simulink model "MSD_4"  (R2021b)
settings: Solver=ode4  StartTime=0.0  StopTime=10.0  FixedStep=0.1  RelTol=1e-3
values from neighbouring files (symbols this model uses):
  A = [0  1; -0.428571428571  0]    [matlab.mat]
  B = [0 0]    [matlab.mat]
  B1 = [0 0.0714285714286]    [matlab.mat]
  B2 = [0.1 0]    [matlab.mat]
  C = [1  0; 0  1]    [matlab.mat]
  D = [0 0]    [matlab.mat]
  F = 1    [matlab.mat]
  k = 6    [matlab.mat]
  m = 14    [matlab.mat]
  x0 = 0.1    [matlab.mat]
settings Model: Creator=jpawl  LastModifiedBy=jpawl

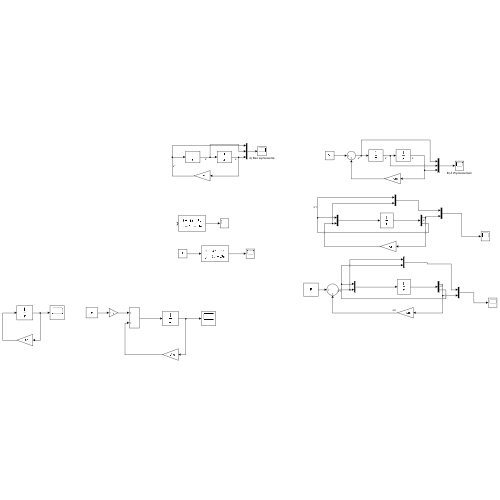
[thumbnail: Simulink's stored preview of the top-level diagram]
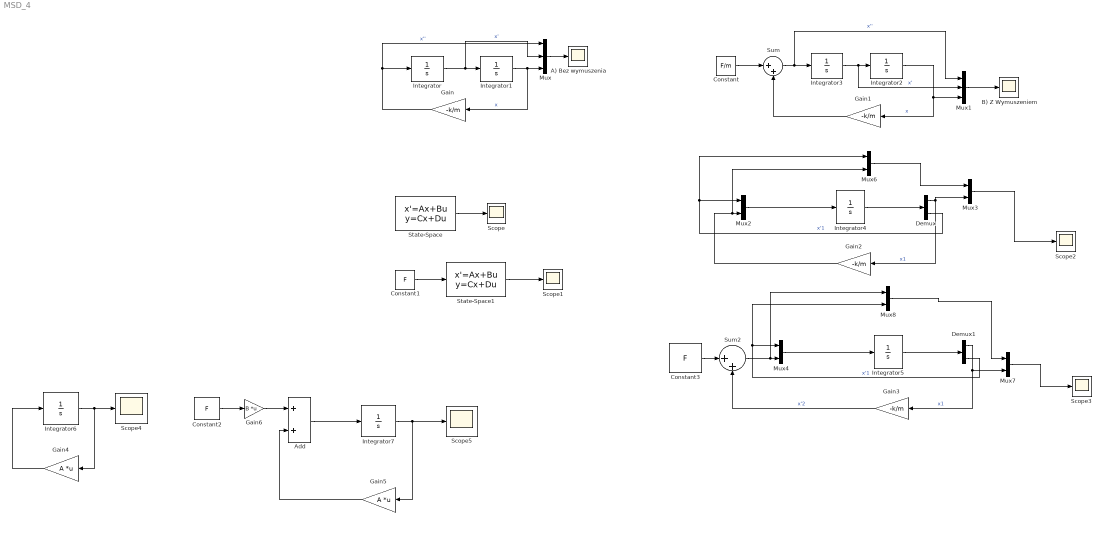
== system MSD_4 ==
  A) Bez wymuszenia : Scope
  Add : Sum
  B) Z Wymuszeniem : Scope
  Constant : Constant  Value=F/m
  Constant1 : Constant  Value=F
  Constant2 : Constant  Value=F
  Constant3 : Constant  Value=F
  Demux : Demux  Outputs=2
  Demux1 : Demux  Outputs=2
  Gain{,1..3} (4 alike) : Gain  Gain=-k/m
  Gain4 : Gain  Gain=A  Multiplication=Matrix(K*u)
  Gain5 : Gain  Gain=A  Multiplication=Matrix(K*u)
  Gain6 : Gain  Gain=B  Multiplication=Matrix(K*u)
  Integrator : Integrator
  Integrator1 : Integrator  InitialCondition=x0
  Integrator2 : Integrator  InitialCondition=x0
  Integrator3 : Integrator
  Integrator4 : Integrator  InitialCondition=B2
  Integrator5 : Integrator  InitialCondition=B2
  Integrator6 : Integrator  InitialCondition=x0
  Integrator7 : Integrator  InitialCondition=B2
  Mux : Mux  Inputs=3
  Mux1 : Mux  Inputs=3
  Mux{2..4,6..8} (6 alike) : Mux  Inputs=2
  Scope{,1..5} (6 alike) : Scope
  State-Space : StateSpace  A=A  B=B  C=C  D=D  InitialCondition=1
  State-Space1 : StateSpace  A=A  B=B1  C=C  D=D  InitialCondition=1
  Sum : Sum  Inputs=|++
  Sum2 : Sum  Inputs=|++
  wires:
  Integrator/1 -> Mux/2, Integrator1/1  "x'"
  Integrator1/1 -> Gain/1, Mux/3  "x"
  Gain/1 -> Mux/1, Integrator/1  "x''"
  Mux/1 -> A) Bez wymuszenia/1
  Constant/1 -> Sum/1
  Sum/1 -> Integrator3/1, Mux1/1  "x''"
  Integrator3/1 -> Integrator2/1, Mux1/2  "x'"
  Integrator2/1 -> Gain1/1, Mux1/3  "x"
  Gain1/1 -> Sum/2
  Mux1/1 -> B) Z Wymuszeniem/1
  State-Space/1 -> Scope/1
  Constant1/1 -> State-Space1/1
  State-Space1/1 -> Scope1/1
  Integrator4/1 -> Demux/1
  Mux2/1 -> Integrator4/1
  Demux/2 -> Mux6/1, Mux2/1  "x'1"
  Demux/1 -> Gain2/1, Mux3/2  "x1"
  Gain2/1 -> Mux6/2, Mux2/2
  Sum2/1 -> Mux8/1, Mux4/2
  Constant3/1 -> Sum2/1
  Demux1/2 -> Mux8/2, Mux4/1  "x'1"
  Integrator5/1 -> Demux1/1
  Demux1/1 -> Mux7/2, Gain3/1  "x1"
  Mux4/1 -> Integrator5/1
  Gain3/1 -> Sum2/2  "x'2"
  Gain4/1 -> Integrator6/1
  Integrator6/1 -> Gain4/1, Scope4/1
  Integrator7/1 -> Gain5/1, Scope5/1
  Gain5/1 -> Add/2
  Constant2/1 -> Gain6/1
  Gain6/1 -> Add/1
  Add/1 -> Integrator7/1
  Mux6/1 -> Mux3/1
  Mux3/1 -> Scope2/1
  Mux8/1 -> Mux7/1
  Mux7/1 -> Scope3/1
